simulink model "scheme1_1"  (R2021a)
settings: Solver=ode1  StartTime=0.0  StopTime=25  FixedStep=Tp  RelTol=1e-3
values from neighbouring files (symbols this model uses):
  k = 6    [exercise1.m]    (also in exercise2.m)
  kp = 1.6    [exercise1.m]    (also in exercise2.m)
  T_1 = 5.9    [exercise1.m]    (also in exercise2.m)
  T_2 = 0.8    [exercise1.m]    (also in exercise2.m)
  Td = 0.08    [exercise1.m]    (also in exercise2.m)
  Ti = 6    [exercise1.m]    (also in exercise2.m)
  Tp = 0.01    [exercise1.m]    (also in exercise2.m)
undefined symbols (not defined in the file or in its folder): magnitude
libraries: pid_lib x1
settings Model: Creator=AgraWoodAdmin  LastModifiedBy=AgraWoodAdmin

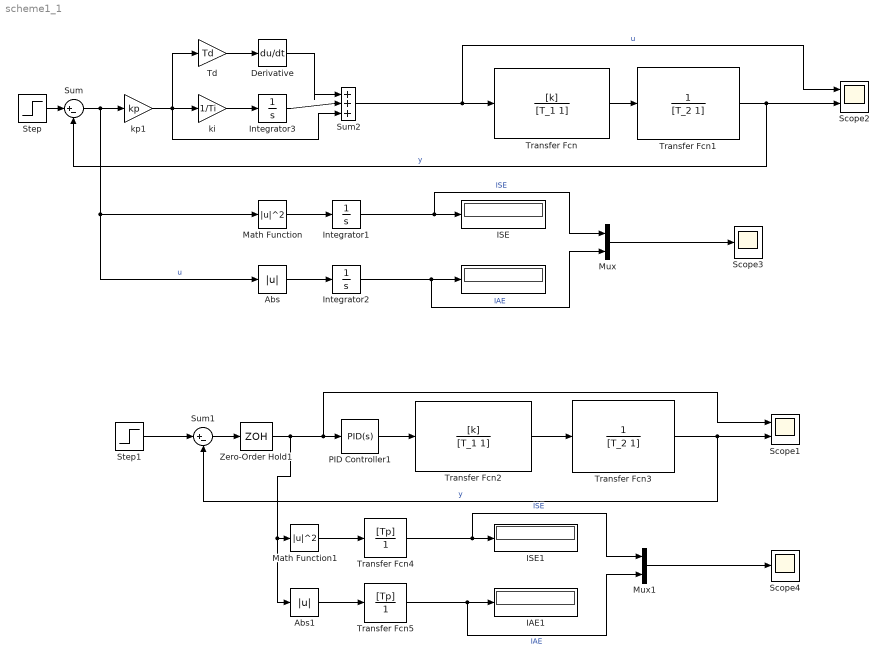
== system scheme1_1 ==
  " " : Display
  Abs : Abs  SaturateOnIntegerOverflow=on
  Abs1 : Abs  SaturateOnIntegerOverflow=on
  Derivative : Derivative
  IAE1 : Display
  ISE : Display
  ISE1 : Display
  Integrator1 : Integrator  InitialCondition=Tp
  Integrator2 : Integrator
  Integrator3 : Integrator
  Math Function : Math  Operator=magnitude^2  SignedPower=on  SaturateOnIntegerOverflow=on
  Math Function1 : Math  Operator=magnitude^2  SignedPower=on  SaturateOnIntegerOverflow=on
  Mux : Mux  Inputs=2
  Mux1 : Mux  Inputs=2
  PID Controller1 : pid_lib/PID Controller  Controller=PID  Form=Parallel  TimeDomain=Continuous-time  UseExternalTs=off  SampleTime=-1  IntegratorMethod=Forward Euler  FilterMethod=Forward Euler  ControllerParametersSource=internal  P=1  I=0.8  D=0.7  UseFilter=on  N=100  TunerSelectOption=Transfer Function Based (PID Tuner App)  InitialConditionSource=internal  InitialConditionForIntegrator=0  InitialConditionForFilter=0  DifferentiatorICPrevScaledInput=0  ExternalReset=none  TrackingMode=off  Kt=1  LimitOutput=off  SatLimitsSource=internal  UpperSaturationLimit=inf  LowerSaturationLimit=-inf  LinearizeAsGain=on  AntiWindupMode=none  Kb=1  POutMin=[]  POutMax=[]  IOutMin=[]  IOutMax=[]  DOutMin=[]  DOutMax=[]  NOutMin=[]  NOutMax=[]  SumOutMin=[]  SumOutMax=[]  SaturationOutMin=[]  SaturationOutMax=[]  PParamMin=[]  PParamMax=[]  IParamMin=[]  IParamMax=[]  DParamMin=[]  DParamMax=[]  NParamMin=[]  NParamMax=[]  KbParamMin=[]  KbParamMax=[]  KtParamMin=[]  KtParamMax=[]  KbOutMin=[]  KbOutMax=[]  KtOutMin=[]  KtOutMax=[]  IntegratorOutMin=[]  IntegratorOutMax=[]  FilterOutMin=[]  FilterOutMax=[]  SumI1OutMin=[]  SumI1OutMax=[]  SumI2OutMin=[]  SumI2OutMax=[]  SumI3OutMin=[]  SumI3OutMax=[]  SumI4OutMin=[]  SumI4OutMax=[]  SumDOutMin=[]  SumDOutMax=[]  DifferentiatorOutMin=[]  DifferentiatorOutMax=[]  FilterDiffOutCoefMin=[]  FilterDiffOutCoefMax=[]  ReciprocalOutMin=[]  ReciprocalOutMax=[]  SumDenOutMin=[]  SumDenOutMax=[]  SumNumOutMin=[]  SumNumOutMax=[]  DivideOutMin=[]  DivideOutMax=[]  UdiffTsProdOutMin=[]  UdiffTsProdOutMax=[]  NTsProdOutMin=[]  NTsProdOutMax=[]  UintegralTsProdOutMin=[]  UintegralTsProdOutMax=[]  UngainTsProdOutMin=[]  UngainTsProdOutMax=[]  IntegratorContinuousStateAttributes=''  IntegratorStateMustResolveToSignalObject=off  IntegratorRTWStateStorageClass=Auto  FilterContinuousStateAttributes=''  FilterStateMustResolveToSignalObject=off  FilterRTWStateStorageClass=Auto  ParallelPVariant=InternalParameters  IdealPVariant=Disabled  IVariant=InternalParameters  DVariant=InternalParameters  IntegratorVariant=Continuous  SatVariant=Disabled  AWVariant=Passthrough  PCopyVariant=Disabled  TRVariant=Disabled  FdbkBlocksVariant=Forward  IdealPFdbkVariant=Disabled  SatFdbkVariant=Disabled  DerivativeFilterVariant=ContFilter  NVariant=InternalParameters  NCopyVariant=Disabled  FilterICVariant=InternalICsFilter  IntegratorICVariant=InternalICs  ExternalResetVariant=Disabled  TRSumVariant=Passthrough  SumFdbkVariant=Disabled  SumVariant=Sum_PID  TsampFilterVariant=InternalTs  TsampNgainVariant=Passthrough  TsampIntegralVariant=Passthrough  ExternalSaturationOutDataTypeStr=Inherit: Same as second input
  Scope1 : Scope  NumInputPorts=2
  Scope2 : Scope  NumInputPorts=2
  Scope3 : Scope
  Scope4 : Scope
  Step : Step  Time=0  SampleTime=Tp
  Step1 : Step  Time=0  SampleTime=Tp
  Sum : Sum  Inputs=|+-
  Sum1 : Sum  Inputs=|+-
  Sum2 : Sum  Inputs=|+++  SaturateOnIntegerOverflow=on
  Td : Gain  Gain=Td  SaturateOnIntegerOverflow=on  OutDataTypeStr=Inherit: Same as input  ParamDataTypeStr=Inherit: Same as input
  Transfer Fcn : TransferFcn  Numerator=[k]  Denominator=[T_1 1]
  Transfer Fcn1 : TransferFcn  Denominator=[T_2 1]
  Transfer Fcn2 : TransferFcn  Numerator=[k]  Denominator=[T_1 1]
  Transfer Fcn3 : TransferFcn  Denominator=[T_2 1]
  Transfer Fcn4 : TransferFcn  Numerator=[Tp]  Denominator=[1]
  Transfer Fcn5 : TransferFcn  Numerator=[Tp]  Denominator=[1]
  Zero-Order Hold1 : ZeroOrderHold  SampleTime=Tp
  ki : Gain  Gain=1/Ti  SaturateOnIntegerOverflow=on  OutDataTypeStr=Inherit: Same as input  ParamDataTypeStr=Inherit: Same as input
  kp1 : Gain  Gain=kp  SaturateOnIntegerOverflow=on  OutDataTypeStr=Inherit: Same as input  ParamDataTypeStr=Inherit: Same as input
  wires:
  Step/1 -> Sum/1
  Transfer Fcn1/1 -> Sum/2, Scope2/2  "y"
  Transfer Fcn/1 -> Transfer Fcn1/1
  PID Controller1/1 -> Transfer Fcn2/1
  Transfer Fcn2/1 -> Transfer Fcn3/1
  Transfer Fcn3/1 -> Scope1/2, Sum1/2  "y"
  Step1/1 -> Sum1/1
  Math Function/1 -> Integrator1/1
  Abs/1 -> Integrator2/1
  Abs1/1 -> Transfer Fcn5/1
  Math Function1/1 -> Transfer Fcn4/1
  Sum1/1 -> Zero-Order Hold1/1
  Integrator2/1 -> Mux/2, " "/1  "IAE"
  Integrator1/1 -> Mux/1, ISE/1  "ISE"
  Sum/1 -> kp1/1, Math Function/1, Abs/1  "u"
  Mux/1 -> Scope3/1
  Mux1/1 -> Scope4/1
  Transfer Fcn4/1 -> Mux1/1, ISE1/1  "ISE"
  Transfer Fcn5/1 -> Mux1/2, IAE1/1  "IAE"
  Zero-Order Hold1/1 -> Abs1/1, Math Function1/1, Scope1/1, PID Controller1/1
  ki/1 -> Integrator3/1
  Integrator3/1 -> Sum2/2
  kp1/1 -> Td/1, Sum2/3, ki/1
  Td/1 -> Derivative/1
  Derivative/1 -> Sum2/1
  Sum2/1 -> Transfer Fcn/1, Scope2/1  "u"
